simulink model "vidcap_video"  (R2018a)
settings: Solver=FixedStepAuto  StartTime=0.0  StopTime=inf  RelTol=1e-3  EnableMultiTasking=on
undefined symbols (not defined in the file): gray, Green, led0, Rec, SDTV, strel
libraries: simulink x4, visionmorphops x2, visiontextngfix x2, dspvision x2, embdlinuxlib x2, visionstatistics x1, visionconversions x1, raspberrypilib x1
settings Model: SimulationMode=external  Creator=migue  LastModifiedBy=migue
settings SolverCC: PositivePriorityOrder=on
settings OptimizationCC: EnhancedBackFolding=on  PassReuseOutputArgsAs=Individual arguments  MaxStackSize=64  OptimizeBlockOrder=speed  DifferentSizesBufferReuse=on  OptimizationCustomize=off
settings DebuggingCC: ParameterTunabilityLossMsg=error
settings HardwareCC: ProdBitPerPointer=32  ProdBitPerSizeT=32  ProdBitPerPtrDiffT=32  ProdLargestAtomicInteger=Long  ProdLargestAtomicFloat=Double  ProdWordSize=32  ProdHWDeviceType=ARM Compatible->ARM Cortex
settings SFSimCC: MATLABDynamicMemAlloc=off
settings RTWCC: SystemTargetFile=ert.tlc  HardwareBoard=Raspberry Pi  TLCOptions="-aInlineSetEventsForThisBaseRateFcn=TLC_FALSE -aSuppressMultiTaskScheduler=TLC_FALSE  -aRateBasedStepFcn=0"  TemplateMakefile=ert_default_tmf  GenerateReport=on  Toolchain=GNU GCC Raspberry Pi  BuildConfiguration=Faster Runs  IncludeHyperlinkInReport=on  LaunchReport=on  GenerateTraceInfo=on  GenerateTraceReport=on  GenerateTraceReportSl=on  GenerateTraceReportSf=on  GenerateTraceReportEml=on
settings CodeAppCC: ForceParamTrailComments=on  IgnoreCustomStorageClasses=off  OperatorAnnotations=on  SimulinkDataObjDesc=on  SFDataObjDesc=on  InsertBlockDesc=on
settings ERTTargetCC: SupportVariableSizeSignals=on

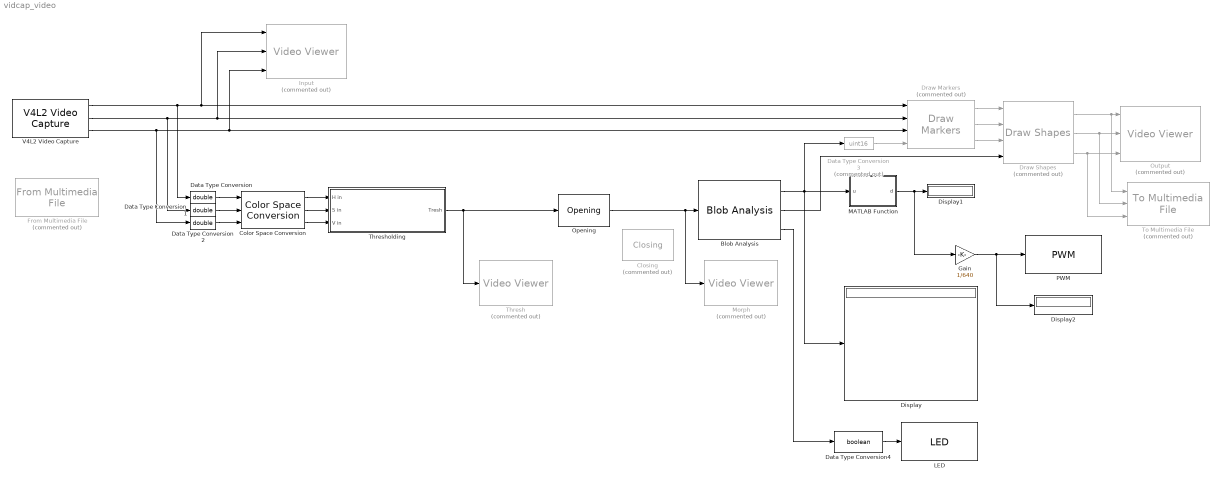
== system vidcap_video ==
  Blob Analysis : visionstatistics/Blob Analysis  Tag=vipblks_row_conv  area=off  centroid=on  bBox=on  majorAxis=off  minorAxis=off  angle=off  eccentricity=off  equivDiameterSq=off  extent=off  perimeter=off  maxBlobs=50  warnIfNumBlobsExceeded=on  isCount=on  useMinArea=on  minArea=500  useMaxArea=off  maxArea=intmax('uint32')  excludeBorderBlob=off  outDT=double  isOutVarDim=off  isFill=on  fillValues=-1  conn=8  isLabel=off  outputMode=Binary point scaling  outputWordLength=32  outputFracLength=16  firstCoeffMode=Binary point scaling  firstCoeffWordLength=16  firstCoeffFracLength=14  secondCoeffMode=Binary point scaling  secondCoeffWordLength=32  secondCoeffFracLength=16  accumMode=Binary point scaling  accumWordLength=32  accumFracLength=0  prodOutputMode=Binary point scaling  prodOutputWordLength=32  prodOutputFracLength=16  roundingMode=Floor  overflowMode=off
      settings: SourceProductName=Computer Vision System Toolbox
  Closing : visionmorphops/Closing  Commented=on  nhoodsrc=Specify via dialog  strel=strel('disk', 11)
      settings: SourceProductName=Computer Vision System Toolbox  SourceProductBaseCode=VP
  Color Space Conversion : visionconversions/Color Space  Conversion  conversion=Obsolete  conversionActive=R'G'B' to HSV  wp_str=D65  rec=Rec. 601 (SDTV)  sys=1125/60/2:1  imagePorts=Separate color signals
      settings: SourceProductName=Computer Vision System Toolbox
  Data Type Conversion : DataTypeConversion  OutDataTypeStr=double
  Data Type Conversion1 : DataTypeConversion  OutDataTypeStr=double
  Data Type Conversion2 : DataTypeConversion  OutDataTypeStr=double
  Data Type Conversion3 : DataTypeConversion  Commented=on  OutDataTypeStr=uint16
  Data Type Conversion4 : DataTypeConversion  OutDataTypeStr=boolean
  Display : Display
  Display1 : Display
  Display2 : Display
  Draw Markers : visiontextngfix/Draw Markers  Commented=on  shape=X-mark  size=10  fill=off  fillClrSource=Specify via dialog  display=White  intensity=200  color=[200 255 100]  opacity=0.6  viewport=Entire image  antialiasing=off  inType=Obsolete  imagePorts=Separate color signals  prodOutputMode=Binary point scaling  prodOutputWordLength=32  prodOutputFracLength=14  memoryMode=Specify word length  memoryWordLength=16  memoryFracLength=15  roundingMode=Floor  overflowMode=off
      settings: SourceProductName=Computer Vision System Toolbox  SourceProductBaseCode=VP
  Draw Shapes : visiontextngfix/Draw Shapes  Commented=on  shape=Rectangles  fill=off  lineWidth=3  fillClrSource=Specify via dialog  display=White  intensity=200  color=[200 255 100]  opacity=0.6  viewport=Entire image  antialiasing=off  inType=Obsolete  imagePorts=Separate color signals  prodOutputMode=Binary point scaling  prodOutputWordLength=32  prodOutputFracLength=14  memoryMode=Specify word length  memoryWordLength=16  memoryFracLength=15  roundingMode=Floor  overflowMode=off
      settings: SourceProductName=Computer Vision System Toolbox
  From Multimedia File : dspvision/From Multimedia File  Commented=on  inputFilename=D:\OneDrive - obf.ateneo.edu\Acads\5th Year\Thesis\Thesis Defense\VID_20190323_150842.mp4  loop=on  numPlays=1  outputStreams=Video only  videoDataType=single  audioDataType=double  inheritSampleTime=on  userDefinedSampleTime=1/30  noAudioOutput=off  isIntensityVideo=off  fourcc=RGB  colorVideoFormat=Separate color signals  outputEOF=off  dataOrg=Column-major  audioFrameSize=1024  computeAudioFrameSize=off  outSamplingMode=Sample based
      settings: SourceProductBaseCode=VP
  Gain : Gain  Gain=1/640
  Input : VideoViewer  Commented=on  imagePorts=separate color signals  colormapValue=gray(256)  FigPos=[1 736 1366 636]
  LED : embdlinuxlib/LED  board=Pi 3 Model B  led=led0 (Green)  blockPlatform=Raspberry Pi
      settings: SourceProductName=Simulink Support Package for Raspberry Pi Hardware  SourceProductBaseCode=RASPPI
  MATLAB Function : MATLAB Function  TreatAsAtomicUnit=on
  Morph : VideoViewer  Commented=on  colormapValue=gray(256)  FigPos=[560 735 796 627]  OpenAtMdlStart=off
  Opening : visionmorphops/Opening  nhoodsrc=Specify via dialog  strel=strel('disk',5)
      settings: SourceProductName=Computer Vision System Toolbox  SourceProductBaseCode=VP
  Output : VideoViewer  Commented=on  imagePorts=separate color signals  colormapValue=gray(256)  FigPos=[-489 776 1366 636]
  PWM : raspberrypilib/PWM  board=Pi 3 Model B  Pin_=21  Frequency=1000  blockPlatform=Raspberry Pi
      settings: SourceProductName=Simulink Support Package for Raspberry Pi Hardware  SourceProductBaseCode=RASPPI
  Thresh : VideoViewer  Commented=on  colormapValue=gray(256)  FigPos=[2 735 681 627]
  Thresholding : Subsystem
  To Multimedia File : dspvision/To Multimedia File  Commented=on  outputFilename=D:\OneDrive\Desktop\HSV Output\output.avi  streamSelection=Video only  videoCompressor=None (uncompressed)  audioCompressor=None (uncompressed)  imagePorts=Separate color signals  fileType=AVI  audioDatatype=Determine from input data type  fourcc=RGB  videoQuality=75  mj2000CompFactor=10
      settings: SourceProductName=Computer Vision System Toolbox  SourceProductBaseCode=VP
  V4L2 Video Capture : embdlinuxlib/V4L2 Video Capture  m_devName='/dev/video0'  roi=[0, 0, 640, 480]  imSizeSelection=640x480  imSize=[640, 480]  pixelFormat=RGB  pixelOrder=Planar  sampleTime=1/30  simOutput=Colorbars  blockPlatform=Raspberry Pi
      settings: SourceProductName=Simulink Support Package for Raspberry Pi Hardware  SourceProductBaseCode=RASPPI
  wires:
  V4L2 Video Capture/1 -> Data Type Conversion/1, Draw Markers/1, Input/1
  V4L2 Video Capture/2 -> Input/2, Draw Markers/2, Data Type Conversion1/1
  V4L2 Video Capture/3 -> Data Type Conversion2/1, Draw Markers/3, Input/3
  Thresholding/1(Tresh) -> Opening/1, Thresh/1
  Opening/1 -> Morph/1, Blob Analysis/1
  Draw Markers/3 -> Draw Shapes/3
  Draw Markers/2 -> Draw Shapes/2
  Draw Markers/1 -> Draw Shapes/1
  Blob Analysis/2 -> Draw Shapes/4
  Draw Shapes/1 -> To Multimedia File/1, Output/1
  Draw Shapes/2 -> Output/2, To Multimedia File/2
  Draw Shapes/3 -> Output/3, To Multimedia File/3
  Color Space Conversion/1 -> Thresholding/1(H in)
  Color Space Conversion/2 -> Thresholding/2(S in)
  Color Space Conversion/3 -> Thresholding/3(V in)
  Blob Analysis/1 -> Display/1, MATLAB Function/1(u), Data Type Conversion3/1
  MATLAB Function/1(d) -> Gain/1, Display1/1
  Data Type Conversion/1 -> Color Space Conversion/1
  Data Type Conversion1/1 -> Color Space Conversion/2
  Data Type Conversion2/1 -> Color Space Conversion/3
  Data Type Conversion3/1 -> Draw Markers/4
  Gain/1 -> Display2/1, PWM/1
  Data Type Conversion4/1 -> LED/1
  Blob Analysis/3 -> Data Type Conversion4/1

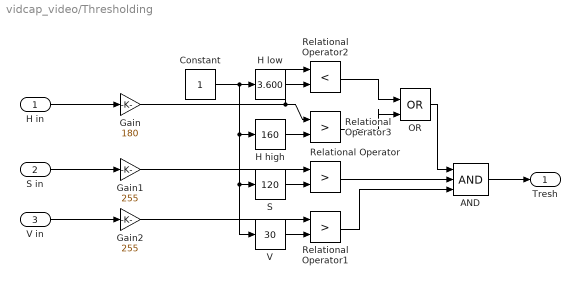
== system vidcap_video/Thresholding ==
  H in : Inport
  S in : Inport  Port=2
  V in : Inport  Port=3
  AND : Logic  Inputs=3  IconShape=distinctive  AllPortsSameDT=off  OutDataTypeStr=boolean
  Constant : Constant
  Gain : Gain  Gain=180
  Gain1 : Gain  Gain=255
  Gain2 : Gain  Gain=255
  H high : simulink/Math Operations/Slider Gain  gain=160  low=0  high=180
  H low : simulink/Math Operations/Slider Gain  gain=3.600  low=0  high=180
  OR : Logic  Operator=OR  IconShape=distinctive  AllPortsSameDT=off  OutDataTypeStr=boolean
  Relational Operator : RelationalOperator  Operator=>  OutDataTypeStr=boolean  RndMeth=Simplest
  Relational Operator1 : RelationalOperator  Operator=>  OutDataTypeStr=boolean  RndMeth=Simplest
  Relational Operator2 : RelationalOperator  Operator=<  OutDataTypeStr=boolean  RndMeth=Simplest
  Relational Operator3 : RelationalOperator  Operator=>  OutDataTypeStr=boolean  RndMeth=Simplest
  S : simulink/Math Operations/Slider Gain  gain=120  low=0  high=255
  V : simulink/Math Operations/Slider Gain  gain=30  low=0  high=255
  Tresh : Outport
  wires:
  Constant/1 -> H low/1, H high/1, V/1, S/1
  Gain2/1 -> Relational Operator1/1
  Relational Operator1/1 -> AND/3
  H in/1 -> Gain/1
  V/1 -> Relational Operator1/2
  Gain1/1 -> Relational Operator/1
  Gain/1 -> Relational Operator3/1, Relational Operator2/1
  Relational Operator3/1 -> OR/2
  AND/1 -> Tresh/1
  H high/1 -> Relational Operator3/2
  H low/1 -> Relational Operator2/2
  S/1 -> Relational Operator/2
  Relational Operator2/1 -> OR/1
  Relational Operator/1 -> AND/2
  OR/1 -> AND/1
  S in/1 -> Gain1/1
  V in/1 -> Gain2/1

== matlab function vidcap_video/MATLAB Function ==
  data: u input; d output
function d = dist(u)
distance = 0;
rc = size(u);
for i=1:rc(1)-1
    for k=i+1:rc(1)
        if u(i,2) > 0 
            if abs(u(i,1) - u(k,1)) < 50
                distance = abs(u(k,2) - u(i,2));
            end
        end
    end
end
d = distance;
